simulink model "toPWM2"  (R2015b)
settings: Solver=VariableStepAuto  StartTime=0.0  StopTime=10.0  RelTol=1e-3
settings Model: Creator=erik  LastModifiedBy=erik

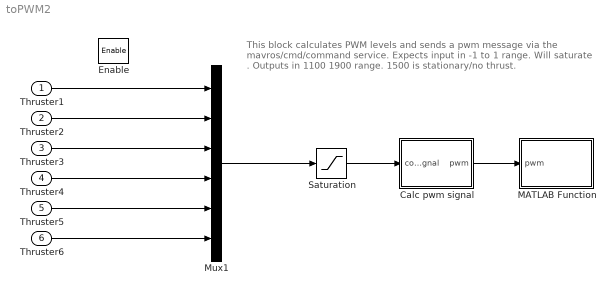
== system toPWM2 ==
  note: This block calculates PWM levels and sends a pwm message
      | via the mavros/cmd/command service.
      |
      | Expects input in -1 to 1 range. Will saturate . Outputs in 1100 1900 range. 1500 is stationary/no thrust.
  Thruster1 : Inport  OutDataTypeStr=single  PortDimensions=6
  Thruster2 : Inport  Port=2  OutDataTypeStr=single  PortDimensions=6
  Thruster3 : Inport  Port=3  OutDataTypeStr=single  PortDimensions=6
  Thruster4 : Inport  Port=4  OutDataTypeStr=single  PortDimensions=6
  Thruster5 : Inport  Port=5  OutDataTypeStr=single  PortDimensions=6
  Thruster6 : Inport  Port=6  OutDataTypeStr=single  PortDimensions=6
  Enable : EnablePort
  Calc pwm signal : MATLAB Function  TreatAsAtomicUnit=on
  MATLAB Function : MATLAB Function  TreatAsAtomicUnit=on
  Mux1 : Mux  Inputs=6
  Saturation : Saturate  UpperLimit=1  LowerLimit=-1
  wires:
  Saturation/1 -> Calc pwm signal/1(controlsignal)
  Thruster1/1 -> Mux1/1
  Mux1/1 -> Saturation/1
  Thruster4/1 -> Mux1/4
  Thruster6/1 -> Mux1/6
  Thruster5/1 -> Mux1/5
  Thruster2/1 -> Mux1/2
  Thruster3/1 -> Mux1/3
  Calc pwm signal/1(pwm) -> MATLAB Function/1(pwm)

== matlab function toPWM2/MATLAB Function ==
  data: pwm input
function  fcn(pwm)
%#codegen
pwm_client = rossvcclient('/mavros/cmd/command');
%create a message
pwm_message=rosmessage('mavros_msgs/CommandLong');
%183 = do_set_servo command 
pwm_message.Command=183;
for i=1:6
    pwm_message.Param1 = i;
    pwm_message.Param2 = pwm(i);
    a=call(pwm_client,pwm_message);
end
end

== matlab function toPWM2/Calc pwm signal ==
  data: controlsignal input; pwm output
function pwm = calcPWM(controlsignal)
 % thruster values should be between 1100 and 1900 microseconds (us)
 % values less than 1500 us are backwards; values more than are forwards

pwm=(controlsignal + 1) * 400 + 1100;

end
